simulink model "VSM_specComp"  (R2024b)
settings: Solver=ode3  StartTime=0.0  StopTime=4  FixedStep=HWSampleTime  RelTol=1e-3
PostLoadFcn:
  | EXEC_MODE=ExecutionMode.SIMULATION;
  | %Sim_TP33_VSM_HSS_init
InitFcn:
  | %EXEC_MODE=ExecutionMode.SIMULATION;
  | %Sim_TP33_VSM_HSS_init
StopFcn:
  | %sim2struct
undefined symbols (not defined in the file): ControlSampleTime, DiscIntNeverNeededParam, fault_dur, Grid, HWSampleTime, LCL, Manage, Param, SM, t_fault, V_DC, VSMCTRL
libraries: FriedrichLibrary x38, simulink x16, TriphaseHardwaremodule x12, spsThreePhaseSeriesRLCBranchLib x4, spsThreePhaseVIMeasurementLib x4, spsThreePhaseBreakerLib x4, spsGroundLib x2, spsUniversalBridgeLib x2, spsVoltageMeasurementLib x2, spsDCVoltageSourceLib x2, spsEdgeDetectorLib x2, spsMeanLib x2
(part 5 of 5)

== system VSM_specComp/VSM_2/VSM1/VSM/CONTROL/VSMOC1/VSMOC/Enabled Subsystem ==
  u_abs : Inport
  Enable : EnablePort
  Out1 : Outport
  wires:
  u_abs/1 -> Out1/1

== system VSM_specComp/VSM_2/VSM1/VSM/CONTROL/VSMOC1/VSMOC/Enabled Subsystem1 ==
  P : Inport
  Enable : EnablePort
  Out1 : Outport
  wires:
  P/1 -> Out1/1

== system VSM_specComp/VSM_2/VSM1/VSM/CONTROL/VSMOC1/VSMOC/FRT Slow Down ==
  U : Inport
  Bias : Bias  Bias=0.2  SaturateOnIntegerOverflow=off
  Complex to Magnitude-Angle : ComplexToMagnitudeAngle
  Demux : Demux  Outputs=2
  Real-Imag to Complex : RealImagToComplex
  Saturation : Saturate  UpperLimit=1  LowerLimit=0
  Terminator : Terminator
  Unit Delay4 : UnitDelay  SampleTime=ControlSampleTime  HasFrameUpgradeWarning=on
  K : Outport  VectorParamsAs1DForOutWhenUnconnected=off
  wires:
  Complex to Magnitude-Angle/1 -> Bias/1
  Demux/2 -> Real-Imag to Complex/2
  Demux/1 -> Real-Imag to Complex/1
  Real-Imag to Complex/1 -> Complex to Magnitude-Angle/1
  U/1 -> Unit Delay4/1
  Complex to Magnitude-Angle/2 -> Terminator/1
  Bias/1 -> Saturation/1
  Saturation/1 -> K/1
  Unit Delay4/1 -> Demux/1

== system VSM_specComp/VSM_2/VSM1/VSM/CONTROL/VSMOC1/VSMOC/Integrator (Angle) ==
  Reset : Inport
  omega : Inport  Port=2
  d_phi0 : Inport  Port=3
  Angle Integrator Reset[SI] : FriedrichLibrary/Discrete Stuff/Angle Integrator Reset[SI]  Ts=ControlSampleTime
  Delay : Delay  DelayLength=1  InitialConditionSource=Input port
      settings: InputPortMap=u0,p4
  Gain3 : Gain  Gain=-1*ControlSampleTime
  Scope : Scope  NumInputPorts=2
  Scope1 : Scope  NumInputPorts=2
  Sum1 : Sum  Inputs=|++
  Sum9 : Sum  Inputs=|+-
  phi : Outport  VectorParamsAs1DForOutWhenUnconnected=off
  wires:
  Gain3/1 -> Sum9/2, Scope/2, Delay/2
  omega/1 -> Gain3/1, Angle Integrator Reset[SI]/2
  Angle Integrator Reset[SI]/1 -> Delay/1, phi/1  "Phi [rad]"
  Reset/1 -> Scope1/1, Angle Integrator Reset[SI]/1
  Sum9/1 -> Sum1/1
  Sum1/1 -> Scope1/2, Angle Integrator Reset[SI]/3
  d_phi0/1 -> Sum9/1
  Delay/1 -> Scope/1, Sum1/2

== system VSM_specComp/VSM_2/VSM1/VSM/CONTROL/VSMOC1/VSMOC/Integrator (Inertia) ==
  dPTa : Inport
  omega0 [pu] : Inport  Port=2
  Enable : EnablePort
  Integrator (inertia) : DiscreteIntegrator  gainval=1  InitialConditionSource=external  InitialCondition=1  SampleTime=ControlSampleTime  ICPrevOutput=DiscIntNeverNeededParam  ICPrevScaledInput=DiscIntNeverNeededParam
  omega [pu] : Outport  VectorParamsAs1DForOutWhenUnconnected=off
  wires:
  omega0 [pu]/1 -> Integrator (inertia)/2
  Integrator (inertia)/1 -> omega [pu]/1  "Omega [pu]"
  dPTa/1 -> Integrator (inertia)/1

== system VSM_specComp/VSM_2/VSM1/VSM/CONTROL/VSMOC1/VSMOC/P Filter Init ==
  Tau : Inport
  dP0 : Inport  Port=2
  Enable : EnablePort  StatesWhenEnabling=reset
  Divide4 : Product  Inputs=*/
  Gain : Gain  Gain=-1
  Integrator1 : DiscreteIntegrator  gainval=1  InitialConditionSource=external  SampleTime=ControlSampleTime  ICPrevOutput=DiscIntNeverNeededParam  ICPrevScaledInput=DiscIntNeverNeededParam
  dP : Outport  VectorParamsAs1DForOutWhenUnconnected=off
  wires:
  dP0/1 -> Integrator1/2
  Gain/1 -> Divide4/1
  Divide4/1 -> Integrator1/1
  Tau/1 -> Divide4/2
  Integrator1/1 -> dP/1, Gain/1

== system VSM_specComp/VSM_2/VSM1/VSM/CONTROL/VSMOC1/VSMOC/Q(U)-PI-Regler ==
  Tau : Inport
  E : Inport  Port=2
  E0 : Inport  Port=3
  Enable : EnablePort  StatesWhenEnabling=reset
  Divide2 : Product  Inputs=*/
  Integrator : DiscreteIntegrator  gainval=1  InitialConditionSource=external  InitialCondition=0.9  SampleTime=ControlSampleTime  ICPrevOutput=DiscIntNeverNeededParam  ICPrevScaledInput=DiscIntNeverNeededParam
  Sum1 : Sum  Inputs=|+-
  E_fil : Outport  VectorParamsAs1DForOutWhenUnconnected=off
  wires:
  E0/1 -> Integrator/2
  Divide2/1 -> Integrator/1
  E/1 -> Sum1/1
  Tau/1 -> Divide2/2
  Integrator/1 -> Sum1/2, E_fil/1  "E [pu]"
  Sum1/1 -> Divide2/1

== system VSM_specComp/VSM_2/VSM1/VSM/CONTROL/VSMOC1/VSMOC/Subsystem ==
  first_run : Inport
  u_dq : Inport  Port=2
  u_dq_pll : Inport  Port=3
  phi_pll : Inport  Port=4
  Enable : EnablePort
  Complex to Magnitude-Angle : ComplexToMagnitudeAngle
  Demux : Demux  Outputs=2
  Real-Imag to Complex : RealImagToComplex
  Switch : Switch  Criteria=u2 > Threshold  SaturateOnIntegerOverflow=off  InputSameDT=off
  Switch1 : Switch  Criteria=u2 ~= 0  SaturateOnIntegerOverflow=off  InputSameDT=off
  "first_run " : InportShadow
  u_abs : Outport  InitialOutput=1  VectorParamsAs1DForOutWhenUnconnected=off
  u_ang : Outport  Port=2  InitialOutput=0  VectorParamsAs1DForOutWhenUnconnected=off
  wires:
  Switch/1 -> u_ang/1
  phi_pll/1 -> Switch/1
  Real-Imag to Complex/1 -> Complex to Magnitude-Angle/1
  Demux/1 -> Real-Imag to Complex/1
  Demux/2 -> Real-Imag to Complex/2
  Complex to Magnitude-Angle/1 -> u_abs/1
  Switch1/1 -> Demux/1
  first_run/1 -> Switch1/2
  u_dq/1 -> Switch1/3
  u_dq_pll/1 -> Switch1/1
  "first_run "/1 -> Switch/2
  Complex to Magnitude-Angle/2 -> Switch/3

== system VSM_specComp/VSM_2/VSM1/VSM/MANAGEMENT/Subsystem1/Subsystem/T->ControlSampleTime ==
  In1 : Inport
  Discrete Derivative : simulink/Discrete/Discrete Derivative  gainval=1.0  ICPrevScaledInput=0.0  OutMin=[]  OutMax=[]  OutDataType=fixdt(1, 16)  OutScaling=2^-10  DoSatur=off
  Out1 : Outport
  wires:
  Discrete Derivative/1 -> Out1/1
  In1/1 -> Discrete Derivative/1

== system VSM_specComp/VSM_2/VSM1/VSM/MANAGEMENT/sp_VSM/RateLimit/ratelimitspPQ ==
  rateup : Inport
  x : Inport  Port=2
  ratedown : Inport  Port=3
  x0 : Inport  Port=4
  Delay : Delay  DelayLength=1  InitialConditionSource=Input port  SampleTime=Ts
      settings: InputPortMap=u0,p4
  Gain : Gain  Gain=Ts
  Gain1 : Gain  Gain=-Ts
  Saturation Dynamic2 : simulink/Discontinuities/Saturation Dynamic  OutMin=[]  OutMax=[]  OutDataTypeStr=Inherit: Same as second input  OutDataType=fixdt(1, 16)  OutScaling=2^-10  DoSatur=off
  Sum : Sum  Inputs=|+-
  Sum1 : Sum  Inputs=|++
  x_slow : Outport  VectorParamsAs1DForOutWhenUnconnected=off
  wires:
  Gain1/1 -> Saturation Dynamic2/3
  ratedown/1 -> Gain1/1
  rateup/1 -> Gain/1
  Gain/1 -> Saturation Dynamic2/1
  x0/1 -> Delay/2
  Sum1/1 -> Delay/1, x_slow/1
  Saturation Dynamic2/1 -> Sum1/1
  Sum/1 -> Saturation Dynamic2/2
  Delay/1 -> Sum/2, Sum1/2
  x/1 -> Sum/1

== matlab function VSM_specComp/VSM_1/VSM1/VSM/MANAGEMENT/Subsystem1/Subsystem/MATLAB Function2 ==
  data: i_inv input; i_sp output; PQ_out input; CC output; i_abs input; der input; set1 output; U_cap input; U_der1 input; U_der2 input
function [i_sp, CC, set1]= fcn(i_inv, PQ_out, i_abs, der, U_cap, U_der1, U_der2)
    persistent set
    if isempty(set)
        set = 0;
    end

    persistent d
    if isempty(d)
        d = 0;
    end    
    
    persistent x
    if isempty(x)
        x = 0;
    end    
    
    persistent i_sp_old
    if isempty(i_sp_old)
        i_sp_old = [0 0];
    end
    
    persistent a
    if isempty(a)
        a = [10 10 10 10];
    end
    
    persistent a_u
    if isempty(a_u)
        a_u = [10 10 10 10];
    end
    
    persistent zero
    if isempty(zero)
        zero = [10 10 10 10];
    end  
    
    persistent time
      if isempty(time)
        time = 0;
      end    
    time = time +1;
    
    persistent regler
    if isempty(regler)
        regler = 0;
    end    
    persistent sdf
    if isempty(sdf)
        sdf = 1;
    end  

    CC = false;
    i_sp = [0 0];
    f = 0;
    adf = 10;
    %i_abs = sqrt(i_inv(1)^2 + i_inv(2)^2 + i_inv(3)^2);
    
    if i_abs >= 1.2 && d == 0 % && U_cap <= 0.9 %momentan hohe Spannung
        CC = true;
        set = 1;
    end
    
    if set == 1
        
      i_sp = [0 0];
   CC = true;
    end
    
    if i_abs <= 1 && set == 1 %&& sum(a>1) <= 1
        
        set = 2;
        
        i_sp_old = [i_inv(1) i_inv(2)];
       CC = true;

    end
    a = [a(2:4) i_abs];
    a_u = [a_u(2:4) PQ_out(2)/U_cap];
    
    if set == 2 %&& sum(a>1) <= 1 %&& sum(a_u>0.4) == 0
        [angle, mag] = cart2pol(i_sp_old(1), i_sp_old(2));
        d = 2;
        if PQ_out(2)/U_cap <=0
            f = 6;
        else
        f = 6*(1 - PQ_out(2)/U_cap);            %%lieber PI benutzen und/oder Faktoren in Abhängigkeit von dU machen
        %f = ( PQ_out(2)/U_cap/0.5)^0.5;
        end
        regler = regler - 0.1*(1 - PQ_out(2)/U_cap)+angle*sdf;
i_sp = [regler, 1];
sdf=0;
     %   regler = regler + 0.98 - PQ_out(2)/U_cap;
%f = regler*0.1;
%         if abs(0-U_der1)<= 0.5
%             zero = [zero(2:4) 0]
%         else
%             zero = [zero(2:4) 10]
%         end
%         
%         if sum(zero) == 0 && U_der2 <0
%             f = 0;
%         end
        
        %i_sp = [angle-1/100*f, 1];
        
        [i_sp(1), i_sp(2)]  = pol2cart(i_sp(1), i_sp(2));
        
%         if sum(zero) == 0 && U_der2 <0
%             set = 3;
%             i_sp = [i_inv(1) i_inv(2)];
%         end
        i_sp_old = i_sp;
        CC = true;
        
%         if U_der2 <= 0 && abs(0-U_der1)<= 0.5
%             
%             f = 0;
%         end
%         


    end
    
%     letzte Bedingung ist ungünstig. Entweder Erfüllung des
%     Stromsollwertes mit i_sp~=0, oder Counter in set 2
    
%     if abs(PQ_out(1)) <= 0.05 && PQ_out(2) > 0 && set == 2 && sqrt(PQ_out(1)^2 + PQ_out(2)^2) > 0.1
%               
%        set = 3
%        
%        %i_sp_old = [i_inv(1) i_inv(2)];          % nimmt den aktuellen Stromwert für Blindstrombestimmung
%         CC = true;
%     end    

    if PQ_out(2)/U_cap >= 0.98 && set == 2 %&& sum(a_u>0.4) == 4 
        %set = 3;
        CC = true;
        adf = 20;
              %  CC = false;
        %set = 0;
       % i_sp_old = [0 0];
    end

    if set == 3
       
     % i_sp = i_sp_old * (1 - U_cap);
      i_sp = i_sp_old * 1;
      %i_sp = [0.28 -1.06];
       CC = true;
x = x +1;

    if x >= 50
        set = 4;
        CC = false;
        x = 0;
        i_sp_old = [0 0];
    end
    end
    
   if 0.115 == time/8000 
        set = 4;
        CC = false;
        x = 0;
        i_sp_old = [0 0];
    end
%     
%     % Regelabweichung nicht sonderlich relevant-> lässt CC nur länger
%     % ausgelöst
%     
%     if set == 3 && abs(der(1)) <= 5 && abs(der(2)) <= 5 && abs(i_inv(1)-i_sp(1)) <= 0.05 && abs(i_inv(2)-i_sp(2)) <= 0.05
%         CC = false;
%         set = 0;
%         i_sp_old = [0 0];
%     end
%     

   
    
    %% Spannungswiederkehr ohne Überstrom
    
%     if U_cap >= 0.9
%         CC = true;
%         set = 5;
%         x= x +1;
%     end
%     
%     if x >= 2
%         CC = false;
%         set = 0;
%         x = 0;
%     end
%     %% Spannungswiederkehr
%     
    if i_abs >= 1.2 && U_cap >= 0.6 && set == 4
        CC = true;
        set = 5;
    end
    
    if set == 5
        
      i_sp = [0 0];
   CC = true;
    end
    
    if i_abs <= 0.8 && set == 5
        
        set = 6;
        
        i_sp_old = [i_inv(1) i_inv(2)];
       CC = true;

    end
    q=0;
    if set == 6
        [angle, mag] = cart2pol(i_sp_old(1), i_sp_old(2));
        
        %if PQ_out(1) <= 0.5
        f = 6*(0.83 - PQ_out(1));            %%lieber PI benutzen und/oder Faktoren in Abhängigkeit von dU machen
        %f = ( PQ_out(2)/U_cap/0.5)^0.5;
        %end
        q = 3*(0.28 - PQ_out(2));
        i_sp = [angle-1/100*f-1/100*q, 0.8];
        
        [i_sp(1), i_sp(2)]  = pol2cart(i_sp(1), i_sp(2));
        
        i_sp_old = i_sp;
        CC = true;     
    end
    
    if time/8000 >= 0.23
                CC = false;
        set = 0;
        i_sp_old = [0 0];
    end
        
% %     letzte Bedingung ist ungünstig. Entweder Erfüllung des
% %     Stromsollwertes mit i_sp~=0, oder Counter in set 2
%     
%     if abs(PQ_out(2)) <= 0.05 && PQ_out(1) > 0 && set == 6 && sqrt(PQ_out(1)^2 + PQ_out(2)^2) > 0.1
%               
%        set = 7
%         CC = true;
%     end    
%    
%     if set == 7
%        
%       i_sp = i_sp_old;
%        CC = true;
%     end
%     
%     % Regelabweichung nicht sonderlich relevant-> lässt CC nur länger
%     % ausgelöst
%     
%     if set == 7 && abs(der(1)) <= 10 && abs(der(2)) <= 10 && abs(i_inv(1)-i_sp(1)) <= 0.05 && abs(i_inv(2)-i_sp(2)) <= 0.05
%         CC = false;
%         set = 0;
%         i_sp_old = [0 0];
%     end
    [angle, mag] = cart2pol(i_sp_old(1), i_sp_old(2));
     set1 = set;%regler; %angle;

== matlab function VSM_specComp/VSM_1/VSM1/VSM/MANAGEMENT/current_watchdog/MATLAB Function ==
  data: abs input; CC output; set input; i output; p input; i_inv input
function [CC, i] = fcn(abs, set, p, i_inv)
CC = false;
i=[0 0]

if abs >= set
    CC = true;
    i=[1 1]
%     if PQ(1)<0.5
%         i=[0 1]
%     end
end

== matlab function VSM_specComp/VSM_2/VSM1/VSM/CONTROL/Subsystem1/MATLAB Function ==
  data: phi_vsm output; I input; L1 input; R1 input; U_i input; U_v output
function [phi_vsm, U_v]  = fcn(I, L1, R1, U_i)

phi_vsm = 0;
U_v = [0 ;0];
I = [I(1); I(2)];
Z = [R1 -L1; L1 R1];
for n = -0.8-1:0.0005:2+1
    phi = n;
rot = [cos(phi) sin(phi); -sin(phi) cos(phi)];
U_v = rot.'*([U_i(1); U_i(2)]+Z*I);
if abs(0-U_v(2,1))<= 0.0005
    phi_vsm = phi;
    U_v;
    break
end
end

== matlab function VSM_specComp/VSM_2/VSM1/VSM/MANAGEMENT/Subsystem1/Subsystem/MATLAB Function1 ==
  data: i_inv input; i_sp output; PQ_out input; CC output; i_abs input; der input; set1 output; U_cap input; i_pq_pre input; i_abs_pre input; u_diff input
function [i_sp, CC, set1]= fcn(i_inv, PQ_out, i_abs, der, U_cap, i_pq_pre, i_abs_pre, u_diff)
    persistent set
    if isempty(set)
        set = 0;
    end

    persistent d
    if isempty(d)
        d = 0;
    end    
    
    persistent x
    if isempty(x)
        x = 0;
    end    
    
    persistent i_sp_old
    if isempty(i_sp_old)
        i_sp_old = [0 0];
    end
    
    persistent a
    if isempty(a)
        a = [10 10 10 10];
    end
    
    persistent a_u
    if isempty(a_u)
        a_u = [10 10 10 10 10 10 10 10 10 10 10 10];
    end
    
    persistent zero
    if isempty(zero)
        zero = [10 10 10 10];
    end  
    
    persistent time
      if isempty(time)
        time = 0;
      end    
    time = time +1;
    
    persistent regler
    if isempty(regler)
        regler = 0;
    end    
    persistent sdf
    if isempty(sdf)
        sdf = 1;
    end  

    CC = false;
    i_sp = [0 0];
    f = 0;
    adf = 10;
    %i_abs = sqrt(i_inv(1)^2 + i_inv(2)^2 + i_inv(3)^2);
    
    if i_abs >= 1.05 && d == 0 % && U_cap <= 0.9 %momentan hohe Spannung
        CC = true;
        set = 1;
    end
    
    if set == 1
        
      i_sp = [0 0];
   CC = true;
    end
    
    if i_abs <= 1 && set == 1 %&& sum(a>1) <= 1
        
        set = 2;
        
        i_sp_old = [i_inv(1) i_inv(2)];
       CC = true;

    end
    a = [a(2:4) i_abs];
    a_u = [a_u(2:12) PQ_out(2)/U_cap];
    
    if set == 2 %&& sum(a>1) <= 1 %&& sum(a_u>0.4) == 0
        [angle, mag] = cart2pol(i_sp_old(1), i_sp_old(2));
        d = 2;
        if PQ_out(2)/U_cap <=0
            f = 6;
        else
        f = 6*(1 - PQ_out(2)/U_cap);            %%lieber PI benutzen und/oder Faktoren in Abhängigkeit von dU machen
        %f = ( PQ_out(2)/U_cap/0.5)^0.5;
        end
        regler = regler - +0.1/2/1.1*(1 - PQ_out(2)/U_cap)+angle*sdf;
i_sp = [regler, 1];
sdf=0;
     %   regler = regler + 0.98 - PQ_out(2)/U_cap;
%f = regler*0.1;
%         if abs(0-U_der1)<= 0.5
%             zero = [zero(2:4) 0]
%         else
%             zero = [zero(2:4) 10]
%         end
%         
%         if sum(zero) == 0 && U_der2 <0
%             f = 0;
%         end
        
        %i_sp = [angle-1/100*f, 1];
        
        [i_sp(1), i_sp(2)]  = pol2cart(i_sp(1), i_sp(2));
        
%         if sum(zero) == 0 && U_der2 <0
%             set = 3;
%             i_sp = [i_inv(1) i_inv(2)];
%         end
        i_sp_old = i_sp;
        CC = true;
        
%         if U_der2 <= 0 && abs(0-U_der1)<= 0.5
%             
%             f = 0;
%         end
%         


    end
    
%     letzte Bedingung ist ungünstig. Entweder Erfüllung des
%     Stromsollwertes mit i_sp~=0, oder Counter in set 2
    
%     if abs(PQ_out(1)) <= 0.05 && PQ_out(2) > 0 && set == 2 && sqrt(PQ_out(1)^2 + PQ_out(2)^2) > 0.1
%               
%        set = 3
%        
%        %i_sp_old = [i_inv(1) i_inv(2)];          % nimmt den aktuellen Stromwert für Blindstrombestimmung
%         CC = true;
%     end    

    if set == 2 && abs(der) <= 5 % PQ_out(2)/U_cap >= 0.99 &&PQ_out(2)/U_cap <= 1.01 && %&& sum(a_u>0.95) == 12 
        %set = 3;
        CC = true;
        adf = 20;
        set = 4;
        CC = false;
        x = 0;
       %i_sp_old = [0 0];
       i_sp_old = [i_inv(1) i_inv(2)];
   %set = 3;
    end

    if set == 3
       
     % i_sp = i_sp_old * (1 - U_cap);
      i_sp = i_sp_old * 1;
      %i_sp = [0.28 -1.06];
       CC = true;
x = x +1;

    if x >= 25*4
        set = 4;
        CC = false;
        x = 0;
        i_sp_old = [0 0];
    end
    end
    
   if 0.115 == time/8000 
        set = 4;
        CC = false;
        x = 0;
        i_sp_old = [0 0];
   end
    
      if set == 4
        set = 4;
        CC = false;
        x = 0;
        i_sp_old = [0 0];
    end
%     
%     % Regelabweichung nicht sonderlich relevant-> lässt CC nur länger
%     % ausgelöst
%     
%     if set == 3 && abs(der(1)) <= 5 && abs(der(2)) <= 5 && abs(i_inv(1)-i_sp(1)) <= 0.05 && abs(i_inv(2)-i_sp(2)) <= 0.05
%         CC = false;
%         set = 0;
%         i_sp_old = [0 0];
%     end
%     

   
    
    %% Spannungswiederkehr ohne Überstrom
    
%     if U_cap >= 0.9
%         CC = true;
%         set = 5;
%         x= x +1;
%     end
%     
%     if x >= 2
%         CC = false;
%         set = 0;
%         x = 0;
%     end
%     %% Spannungswiederkehr
%     
    if i_abs >= 1.05 && U_cap >= 0.6 && set == 4
        CC = true;
        set = 5;
    end
    
    if u_diff >= 0.1 && set ==4 && U_cap >= 0.9
        set = 5;
    end
    
    if set == 5
        
      i_sp = [0 0];
   CC = true;
    end

    if i_abs <= 1 && set == 5 %&&i_abs <= i_abs_pre
        
        set = 6;
        
        i_sp_old = [i_inv(1) i_inv(2)];
       CC = true;

    end
    q=0;
    f=0;
%     if set == 6  %% für gleiches P und Q bei gleicher Stromzeigerlänge
%         [angle, mag] = cart2pol(i_sp_old(1), i_sp_old(2));
%         
%         f = 6*(PQ_pre(1) - PQ_out(1));            %%lieber PI benutzen und/oder Faktoren in Abhängigkeit von dU machen
%         q = 6*(PQ_pre(2) - PQ_out(2));
%         i_sp = [angle-1/100*f-1/100*q, 0.92];
%         
%         [i_sp(1), i_sp(2)]  = pol2cart(i_sp(1), i_sp(2));
%         
%         i_sp_old = i_sp;
%         CC = true;     
%     end
        if set == 6  %% für gleichen Wirkstrom und Blindstrom
        [angle, mag] = cart2pol(i_sp_old(1), i_sp_old(2));
        q = 2/2*2*(i_pq_pre(2) - PQ_out(2)/U_cap);          %sorgt dafür, dass in den richtigen Quadranten gezogen wird
        f = 1/2*2*(i_pq_pre(1) - PQ_out(1)/U_cap);           
        i_sp = [angle-1/100*f-1/100*q, i_abs_pre];
        
        [i_sp(1), i_sp(2)]  = pol2cart(i_sp(1), i_sp(2));
        
        i_sp_old = i_sp;
        CC = true;     
    end

    if PQ_out(1)/U_cap >= i_pq_pre(1)-0.01 &&PQ_out(1)/U_cap <= i_pq_pre(1)+0.01 && set == 6 && abs(der) <= 2%time/8000 >= 0.23
                CC = false;
        set = 0;
        i_sp_old = [0 0];
    end
        
% %     letzte Bedingung ist ungünstig. Entweder Erfüllung des
% %     Stromsollwertes mit i_sp~=0, oder Counter in set 2
%     
%     if abs(PQ_out(2)) <= 0.05 && PQ_out(1) > 0 && set == 6 && sqrt(PQ_out(1)^2 + PQ_out(2)^2) > 0.1
%               
%        set = 7
%         CC = true;
%     end    
%    
%     if set == 7
%        
%       i_sp = i_sp_old;
%        CC = true;
%     end
%     
%     % Regelabweichung nicht sonderlich relevant-> lässt CC nur länger
%     % ausgelöst
%     
%     if set == 7 && abs(der(1)) <= 10 && abs(der(2)) <= 10 && abs(i_inv(1)-i_sp(1)) <= 0.05 && abs(i_inv(2)-i_sp(2)) <= 0.05
%         CC = false;
%         set = 0;
%         i_sp_old = [0 0];
%     end
    [angle, mag] = cart2pol(i_sp_old(1), i_sp_old(2));
     set1 = angle;%regler; %angle;

== matlab function VSM_specComp/VSM_2/VSM1/VSM/MANAGEMENT/Subsystem1/Subsystem/MATLAB Function2 ==
  data: i_inv input; i_sp output; PQ_out input; CC output; i_abs input; der input; set1 output; U_cap input; U_der1 input; U_der2 input
function [i_sp, CC, set1]= fcn(i_inv, PQ_out, i_abs, der, U_cap, U_der1, U_der2)
    persistent set
    if isempty(set)
        set = 0;
    end

    persistent d
    if isempty(d)
        d = 0;
    end    
    
    persistent x
    if isempty(x)
        x = 0;
    end    
    
    persistent i_sp_old
    if isempty(i_sp_old)
        i_sp_old = [0 0];
    end
    
    persistent a
    if isempty(a)
        a = [10 10 10 10];
    end
    
    persistent a_u
    if isempty(a_u)
        a_u = [10 10 10 10];
    end
    
    persistent zero
    if isempty(zero)
        zero = [10 10 10 10];
    end  
    
    persistent time
      if isempty(time)
        time = 0;
      end    
    time = time +1;
    
    persistent regler
    if isempty(regler)
        regler = 0;
    end    
    persistent sdf
    if isempty(sdf)
        sdf = 1;
    end  

    CC = false;
    i_sp = [0 0];
    f = 0;
    adf = 10;
    %i_abs = sqrt(i_inv(1)^2 + i_inv(2)^2 + i_inv(3)^2);
    
    if i_abs >= 1.2 && d == 0 % && U_cap <= 0.9 %momentan hohe Spannung
        CC = true;
        set = 1;
    end
    
    if set == 1
        
      i_sp = [0 0];
   CC = true;
    end
    
    if i_abs <= 1 && set == 1 %&& sum(a>1) <= 1
        
        set = 2;
        
        i_sp_old = [i_inv(1) i_inv(2)];
       CC = true;

    end
    a = [a(2:4) i_abs];
    a_u = [a_u(2:4) PQ_out(2)/U_cap];
    
    if set == 2 %&& sum(a>1) <= 1 %&& sum(a_u>0.4) == 0
        [angle, mag] = cart2pol(i_sp_old(1), i_sp_old(2));
        d = 2;
        if PQ_out(2)/U_cap <=0
            f = 6;
        else
        f = 6*(1 - PQ_out(2)/U_cap);            %%lieber PI benutzen und/oder Faktoren in Abhängigkeit von dU machen
        %f = ( PQ_out(2)/U_cap/0.5)^0.5;
        end
        regler = regler - 0.1*(1 - PQ_out(2)/U_cap)+angle*sdf;
i_sp = [regler, 1];
sdf=0;
     %   regler = regler + 0.98 - PQ_out(2)/U_cap;
%f = regler*0.1;
%         if abs(0-U_der1)<= 0.5
%             zero = [zero(2:4) 0]
%         else
%             zero = [zero(2:4) 10]
%         end
%         
%         if sum(zero) == 0 && U_der2 <0
%             f = 0;
%         end
        
        %i_sp = [angle-1/100*f, 1];
        
        [i_sp(1), i_sp(2)]  = pol2cart(i_sp(1), i_sp(2));
        
%         if sum(zero) == 0 && U_der2 <0
%             set = 3;
%             i_sp = [i_inv(1) i_inv(2)];
%         end
        i_sp_old = i_sp;
        CC = true;
        
%         if U_der2 <= 0 && abs(0-U_der1)<= 0.5
%             
%             f = 0;
%         end
%         


    end
    
%     letzte Bedingung ist ungünstig. Entweder Erfüllung des
%     Stromsollwertes mit i_sp~=0, oder Counter in set 2
    
%     if abs(PQ_out(1)) <= 0.05 && PQ_out(2) > 0 && set == 2 && sqrt(PQ_out(1)^2 + PQ_out(2)^2) > 0.1
%               
%        set = 3
%        
%        %i_sp_old = [i_inv(1) i_inv(2)];          % nimmt den aktuellen Stromwert für Blindstrombestimmung
%         CC = true;
%     end    

    if PQ_out(2)/U_cap >= 0.98 && set == 2 %&& sum(a_u>0.4) == 4 
        %set = 3;
        CC = true;
        adf = 20;
              %  CC = false;
        %set = 0;
       % i_sp_old = [0 0];
    end

    if set == 3
       
     % i_sp = i_sp_old * (1 - U_cap);
      i_sp = i_sp_old * 1;
      %i_sp = [0.28 -1.06];
       CC = true;
x = x +1;

    if x >= 50
        set = 4;
        CC = false;
        x = 0;
        i_sp_old = [0 0];
    end
    end
    
   if 0.115 == time/8000 
        set = 4;
        CC = false;
        x = 0;
        i_sp_old = [0 0];
    end
%     
%     % Regelabweichung nicht sonderlich relevant-> lässt CC nur länger
%     % ausgelöst
%     
%     if set == 3 && abs(der(1)) <= 5 && abs(der(2)) <= 5 && abs(i_inv(1)-i_sp(1)) <= 0.05 && abs(i_inv(2)-i_sp(2)) <= 0.05
%         CC = false;
%         set = 0;
%         i_sp_old = [0 0];
%     end
%     

   
    
    %% Spannungswiederkehr ohne Überstrom
    
%     if U_cap >= 0.9
%         CC = true;
%         set = 5;
%         x= x +1;
%     end
%     
%     if x >= 2
%         CC = false;
%         set = 0;
%         x = 0;
%     end
%     %% Spannungswiederkehr
%     
    if i_abs >= 1.2 && U_cap >= 0.6 && set == 4
        CC = true;
        set = 5;
    end
    
    if set == 5
        
      i_sp = [0 0];
   CC = true;
    end
    
    if i_abs <= 0.8 && set == 5
        
        set = 6;
        
        i_sp_old = [i_inv(1) i_inv(2)];
       CC = true;

    end
    q=0;
    if set == 6
        [angle, mag] = cart2pol(i_sp_old(1), i_sp_old(2));
        
        %if PQ_out(1) <= 0.5
        f = 6*(0.83 - PQ_out(1));            %%lieber PI benutzen und/oder Faktoren in Abhängigkeit von dU machen
        %f = ( PQ_out(2)/U_cap/0.5)^0.5;
        %end
        q = 3*(0.28 - PQ_out(2));
        i_sp = [angle-1/100*f-1/100*q, 0.8];
        
        [i_sp(1), i_sp(2)]  = pol2cart(i_sp(1), i_sp(2));
        
        i_sp_old = i_sp;
        CC = true;     
    end
    
    if time/8000 >= 0.23
                CC = false;
        set = 0;
        i_sp_old = [0 0];
    end
        
% %     letzte Bedingung ist ungünstig. Entweder Erfüllung des
% %     Stromsollwertes mit i_sp~=0, oder Counter in set 2
%     
%     if abs(PQ_out(2)) <= 0.05 && PQ_out(1) > 0 && set == 6 && sqrt(PQ_out(1)^2 + PQ_out(2)^2) > 0.1
%               
%        set = 7
%         CC = true;
%     end    
%    
%     if set == 7
%        
%       i_sp = i_sp_old;
%        CC = true;
%     end
%     
%     % Regelabweichung nicht sonderlich relevant-> lässt CC nur länger
%     % ausgelöst
%     
%     if set == 7 && abs(der(1)) <= 10 && abs(der(2)) <= 10 && abs(i_inv(1)-i_sp(1)) <= 0.05 && abs(i_inv(2)-i_sp(2)) <= 0.05
%         CC = false;
%         set = 0;
%         i_sp_old = [0 0];
%     end
    [angle, mag] = cart2pol(i_sp_old(1), i_sp_old(2));
     set1 = set;%regler; %angle;

== matlab function VSM_specComp/VSM_2/VSM1/VSM/MANAGEMENT/current_watchdog/MATLAB Function ==
  data: abs input; CC output; set input; i output; p input; i_inv input
function [CC, i] = fcn(abs, set, p, i_inv)
CC = false;
i=[0 0]

if abs >= set
    CC = true;
    i=[1 1]
%     if PQ(1)<0.5
%         i=[0 1]
%     end
end

== matlab function VSM_specComp/VSM_1/VSM1/VSM/CONTROL/Subsystem1/MATLAB Function ==
  data: phi_vsm output; I input; L1 input; R1 input; U_i input; U_v output
function [phi_vsm, U_v]  = fcn(I, L1, R1, U_i)

phi_vsm = 0;
U_v = [0 ;0];
I = [I(1); I(2)];
Z = [R1 -L1; L1 R1];
for n = -0.8-1:0.0005:2+1
    phi = n;
rot = [cos(phi) sin(phi); -sin(phi) cos(phi)];
U_v = rot.'*([U_i(1); U_i(2)]+Z*I);
if abs(0-U_v(2,1))<= 0.0005
    phi_vsm = phi;
    U_v;
    break
end
end

== matlab function VSM_specComp/VSM_1/VSM1/VSM/MANAGEMENT/Subsystem1/Subsystem/MATLAB Function1 ==
  data: i_inv input; i_sp output; PQ_out input; CC output; i_abs input; der input; set1 output; U_cap input; i_pq_pre input; i_abs_pre input; u_diff input
function [i_sp, CC, set1]= fcn(i_inv, PQ_out, i_abs, der, U_cap, i_pq_pre, i_abs_pre, u_diff)
    persistent set
    if isempty(set)
        set = 0;
    end

    persistent d
    if isempty(d)
        d = 0;
    end    
    
    persistent x
    if isempty(x)
        x = 0;
    end    
    
    persistent i_sp_old
    if isempty(i_sp_old)
        i_sp_old = [0 0];
    end
    
    persistent a
    if isempty(a)
        a = [10 10 10 10];
    end
    
    persistent a_u
    if isempty(a_u)
        a_u = [10 10 10 10 10 10 10 10 10 10 10 10];
    end
    
    persistent zero
    if isempty(zero)
        zero = [10 10 10 10];
    end  
    
    persistent time
      if isempty(time)
        time = 0;
      end    
    time = time +1;
    
    persistent regler
    if isempty(regler)
        regler = 0;
    end    
    persistent sdf
    if isempty(sdf)
        sdf = 1;
    end  

    CC = false;
    i_sp = [0 0];
    f = 0;
    adf = 10;
    %i_abs = sqrt(i_inv(1)^2 + i_inv(2)^2 + i_inv(3)^2);
    
    if i_abs >= 1.05 && d == 0 % && U_cap <= 0.9 %momentan hohe Spannung
        CC = true;
        set = 1;
    end
    
    if set == 1
        
      i_sp = [0 0];
   CC = true;
    end
    
    if i_abs <= 1 && set == 1 %&& sum(a>1) <= 1
        
        set = 2;
        
        i_sp_old = [i_inv(1) i_inv(2)];
       CC = true;

    end
    a = [a(2:4) i_abs];
    a_u = [a_u(2:12) PQ_out(2)/U_cap];
    
    if set == 2 %&& sum(a>1) <= 1 %&& sum(a_u>0.4) == 0
        [angle, mag] = cart2pol(i_sp_old(1), i_sp_old(2));
        d = 2;
        if PQ_out(2)/U_cap <=0
            f = 6;
        else
        f = 6*(1 - PQ_out(2)/U_cap);            %%lieber PI benutzen und/oder Faktoren in Abhängigkeit von dU machen
        %f = ( PQ_out(2)/U_cap/0.5)^0.5;
        end
        regler = regler - +0.1/2/1.1*(1 - PQ_out(2)/U_cap)+angle*sdf;
i_sp = [regler, 1];
sdf=0;
     %   regler = regler + 0.98 - PQ_out(2)/U_cap;
%f = regler*0.1;
%         if abs(0-U_der1)<= 0.5
%             zero = [zero(2:4) 0]
%         else
%             zero = [zero(2:4) 10]
%         end
%         
%         if sum(zero) == 0 && U_der2 <0
%             f = 0;
%         end
        
        %i_sp = [angle-1/100*f, 1];
        
        [i_sp(1), i_sp(2)]  = pol2cart(i_sp(1), i_sp(2));
        
%         if sum(zero) == 0 && U_der2 <0
%             set = 3;
%             i_sp = [i_inv(1) i_inv(2)];
%         end
        i_sp_old = i_sp;
        CC = true;
        
%         if U_der2 <= 0 && abs(0-U_der1)<= 0.5
%             
%             f = 0;
%         end
%         


    end
    
%     letzte Bedingung ist ungünstig. Entweder Erfüllung des
%     Stromsollwertes mit i_sp~=0, oder Counter in set 2
    
%     if abs(PQ_out(1)) <= 0.05 && PQ_out(2) > 0 && set == 2 && sqrt(PQ_out(1)^2 + PQ_out(2)^2) > 0.1
%               
%        set = 3
%        
%        %i_sp_old = [i_inv(1) i_inv(2)];          % nimmt den aktuellen Stromwert für Blindstrombestimmung
%         CC = true;
%     end    

    if set == 2 && abs(der) <= 5 % PQ_out(2)/U_cap >= 0.99 &&PQ_out(2)/U_cap <= 1.01 && %&& sum(a_u>0.95) == 12 
        %set = 3;
        CC = true;
        adf = 20;
        set = 4;
        CC = false;
        x = 0;
       %i_sp_old = [0 0];
       i_sp_old = [i_inv(1) i_inv(2)];
   %set = 3;
    end

    if set == 3
       
     % i_sp = i_sp_old * (1 - U_cap);
      i_sp = i_sp_old * 1;
      %i_sp = [0.28 -1.06];
       CC = true;
x = x +1;

    if x >= 25*4
        set = 4;
        CC = false;
        x = 0;
        i_sp_old = [0 0];
    end
    end
    
   if 0.115 == time/8000 
        set = 4;
        CC = false;
        x = 0;
        i_sp_old = [0 0];
   end
    
      if set == 4
        set = 4;
        CC = false;
        x = 0;
        i_sp_old = [0 0];
    end
%     
%     % Regelabweichung nicht sonderlich relevant-> lässt CC nur länger
%     % ausgelöst
%     
%     if set == 3 && abs(der(1)) <= 5 && abs(der(2)) <= 5 && abs(i_inv(1)-i_sp(1)) <= 0.05 && abs(i_inv(2)-i_sp(2)) <= 0.05
%         CC = false;
%         set = 0;
%         i_sp_old = [0 0];
%     end
%     

   
    
    %% Spannungswiederkehr ohne Überstrom
    
%     if U_cap >= 0.9
%         CC = true;
%         set = 5;
%         x= x +1;
%     end
%     
%     if x >= 2
%         CC = false;
%         set = 0;
%         x = 0;
%     end
%     %% Spannungswiederkehr
%     
    if i_abs >= 1.05 && U_cap >= 0.6 && set == 4
        CC = true;
        set = 5;
    end
    
    if u_diff >= 0.1 && set ==4 && U_cap >= 0.9
        set = 5;
    end
    
    if set == 5
        
      i_sp = [0 0];
   CC = true;
    end

    if i_abs <= 1 && set == 5 %&&i_abs <= i_abs_pre
        
        set = 6;
        
        i_sp_old = [i_inv(1) i_inv(2)];
       CC = true;

    end
    q=0;
    f=0;
%     if set == 6  %% für gleiches P und Q bei gleicher Stromzeigerlänge
%         [angle, mag] = cart2pol(i_sp_old(1), i_sp_old(2));
%         
%         f = 6*(PQ_pre(1) - PQ_out(1));            %%lieber PI benutzen und/oder Faktoren in Abhängigkeit von dU machen
%         q = 6*(PQ_pre(2) - PQ_out(2));
%         i_sp = [angle-1/100*f-1/100*q, 0.92];
%         
%         [i_sp(1), i_sp(2)]  = pol2cart(i_sp(1), i_sp(2));
%         
%         i_sp_old = i_sp;
%         CC = true;     
%     end
        if set == 6  %% für gleichen Wirkstrom und Blindstrom
        [angle, mag] = cart2pol(i_sp_old(1), i_sp_old(2));
        q = 2/2*2*(i_pq_pre(2) - PQ_out(2)/U_cap);          %sorgt dafür, dass in den richtigen Quadranten gezogen wird
        f = 1/2*2*(i_pq_pre(1) - PQ_out(1)/U_cap);           
        i_sp = [angle-1/100*f-1/100*q, i_abs_pre];
        
        [i_sp(1), i_sp(2)]  = pol2cart(i_sp(1), i_sp(2));
        
        i_sp_old = i_sp;
        CC = true;     
    end

    if PQ_out(1)/U_cap >= i_pq_pre(1)-0.01 &&PQ_out(1)/U_cap <= i_pq_pre(1)+0.01 && set == 6 && abs(der) <= 2%time/8000 >= 0.23
                CC = false;
        set = 0;
        i_sp_old = [0 0];
    end
        
% %     letzte Bedingung ist ungünstig. Entweder Erfüllung des
% %     Stromsollwertes mit i_sp~=0, oder Counter in set 2
%     
%     if abs(PQ_out(2)) <= 0.05 && PQ_out(1) > 0 && set == 6 && sqrt(PQ_out(1)^2 + PQ_out(2)^2) > 0.1
%               
%        set = 7
%         CC = true;
%     end    
%    
%     if set == 7
%        
%       i_sp = i_sp_old;
%        CC = true;
%     end
%     
%     % Regelabweichung nicht sonderlich relevant-> lässt CC nur länger
%     % ausgelöst
%     
%     if set == 7 && abs(der(1)) <= 10 && abs(der(2)) <= 10 && abs(i_inv(1)-i_sp(1)) <= 0.05 && abs(i_inv(2)-i_sp(2)) <= 0.05
%         CC = false;
%         set = 0;
%         i_sp_old = [0 0];
%     end
    [angle, mag] = cart2pol(i_sp_old(1), i_sp_old(2));
     set1 = angle;%regler; %angle;
